simulink model "etc_PI_singletasking"  (R2022b)
settings: Solver=FixedStepAuto  StartTime=0.0  StopTime=2.5  RelTol=1e-3
PreLoadFcn:
  | % Controller parameters
  | Kp = 0.3;  % Proportional gain
  | Ki = 2;    % Integral gain
  | Ts = 0.01; % Sample time
settings Model: Creator=jrivitus  LastModifiedBy=bensweet
settings SolverCC: AlgebraicLoopSolver=TrustRegion
settings DataIOCC: LimitDataPoints=on  ReturnWorkspaceOutputs=off
settings OptimizationCC: ExpressionDepthLimit=2147483647  InitFltsAndDblsToZero=on  LifeSpan=1  EfficientTunableParamExpr=on
settings DebuggingCC: UnconnectedInputMsg=warning  UnconnectedOutputMsg=warning  UnconnectedLineMsg=warning  PregeneratedLibrarySubsystemCodeDiagnostic=none  SFMachineParentedDataDiag=warning
settings HardwareCC: ProdBitPerPointer=32  ProdBitPerSizeT=32  ProdBitPerPtrDiffT=32  ProdLargestAtomicFloat=None  ProdIntDivRoundTo=Undefined  ProdEndianess=Unspecified  ProdWordSize=32  ProdHWDeviceType=32-bit Generic
settings ModelReferenceCC: EnableRefExpFcnMdlSchedulingChecks=on  PropagateSignalLabelsOutOfModel=off
settings SFSimCC: SimUseLocalCustomCode=off  MATLABDynamicMemAlloc=off
settings RTWCC: Description=Real-Time Workshop Embedded Coder (no auto configuration)  SystemTargetFile=ert.tlc  GenCodeOnly=on  TemplateMakefile=ert_default_tmf  GenerateReport=on  RTWUseLocalCustomCode=off  IncludeHyperlinkInReport=on  LaunchReport=on  GenerateTraceInfo=on  DLArmComputeVersion=19.05
settings CodeAppCC: IgnoreCustomStorageClasses=off  CustomSymbolStrType=$N$R$M  StateflowObjectComments=on  InternalIdentifier=Classic
settings ERTTargetCC: MultiwordLength=2048  GenerateSampleERTMain=on  SupportContinuousTime=on  ERTCustomFileTemplate=example_file_process.tlc  ConvertIfToSwitch=off  SuppressUnreachableDefaultCases=off
settings ConfigComp: CovMetricSettings=dw  CovSaveCumulativeToWorkspaceVar=on  CovSaveSingleToWorkspaceVar=on  CovExternalEMLEnable=off  CovSFcnEnable=off

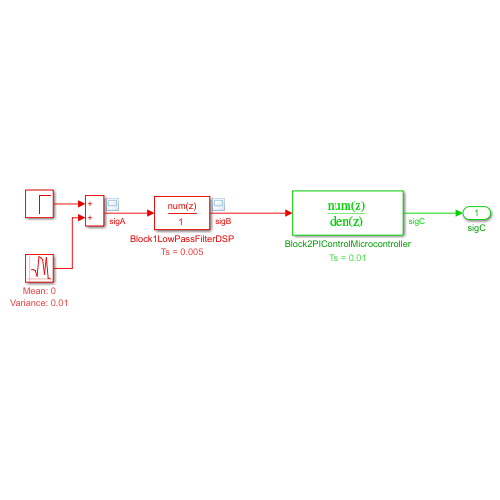
[thumbnail: Simulink's stored preview of the top-level diagram]
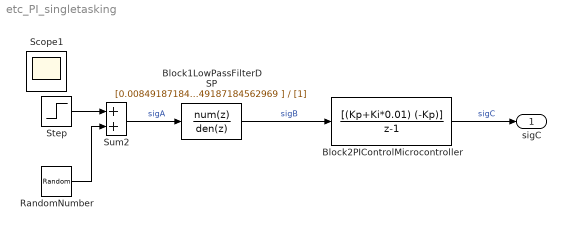
== system etc_PI_singletasking ==
  Block1LowPassFilterDSP : DiscreteFilter  Numerator=|  Denominator=[1]  SampleTime=0.005
      | [0.00849187184562969	0.0444846983267221	0.117299133563462	0.199122538167043	0.235872521380986	0.199122538167043	0.117299133563462	0.0444846983267221	0.00849187184562969
      | ]
      settings: AttributesFormatString=Ts = %<SampleTime>
  Block2PIControlMicrocontroller : DiscreteTransferFcn  Numerator=[(Kp+Ki*0.01) (-Kp)]  Denominator=[1 -1]  SampleTime=0.01
      settings: AttributesFormatString=Ts = %<SampleTime>
  RandomNumber : RandomNumber  Variance=0.01  SampleTime=0.005
      settings: AttributesFormatString=Mean: %<Mean>\nVariance: %<Variance>
  Step : Step  SampleTime=0.005
  Sum2 : Sum  InputSameDT=on  SaturateOnIntegerOverflow=on  OutDataTypeStr=Inherit: Same as first input
  sigC : Outport  VectorParamsAs1DForOutWhenUnconnected=off
  Scope1 : Scope
  wires:
  Sum2/1 -> Block1LowPassFilterDSP/1  "sigA"
  Step/1 -> Sum2/1
  RandomNumber/1 -> Sum2/2
  Block2PIControlMicrocontroller/1 -> sigC/1  "sigC"
  Block1LowPassFilterDSP/1 -> Block2PIControlMicrocontroller/1  "sigB"
